simulink model "twoarealfc"  (R2025a)
settings: Solver=VariableStepAuto  StartTime=0.0  StopTime=10  RelTol=1e-3
settings Model: Creator=Lijoofficial  LastModifiedBy=Lijoofficial

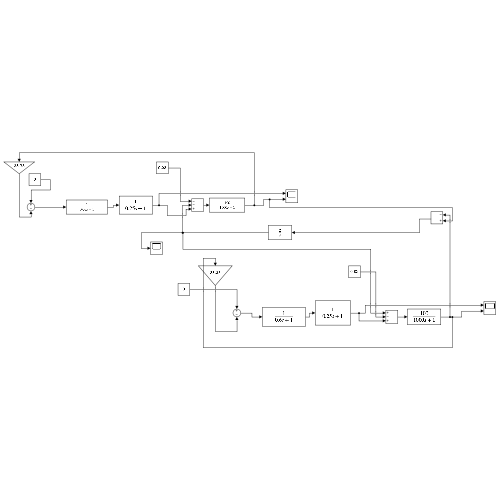
[thumbnail: Simulink's stored preview of the top-level diagram]
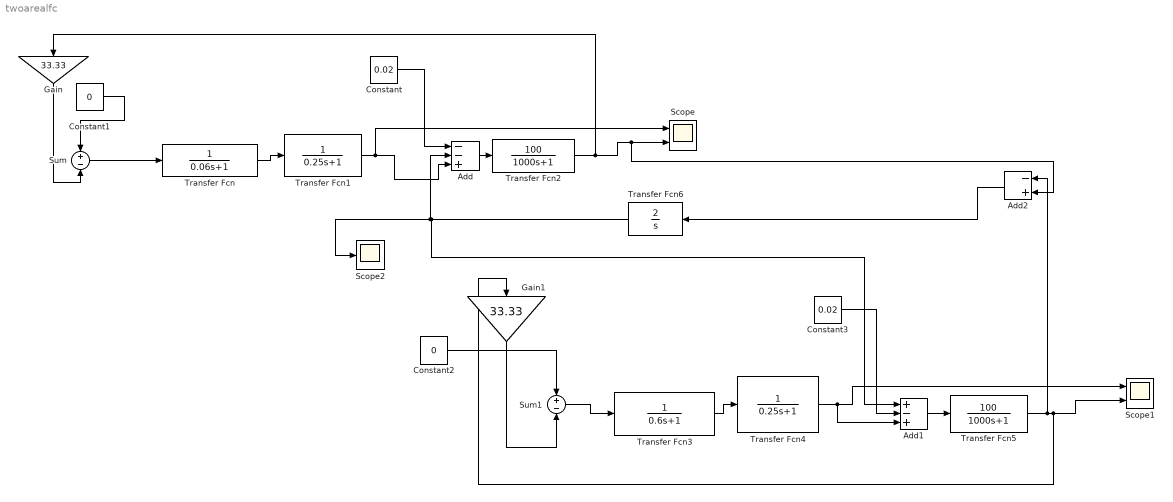
== system twoarealfc ==
  Add : Sum  Inputs=--+
  Add1 : Sum  Inputs=+-+
  Add2 : Sum  Inputs=-+
  Constant : Constant  Value=0.02
  Constant1 : Constant  Value=0
  Constant2 : Constant  Value=0
  Constant3 : Constant  Value=0.02
  Gain : Gain  Gain=33.33
  Gain1 : Gain  Gain=33.33
  Scope : Scope  NumInputPorts=2
      settings: ActiveDisplayYMinimum=-0.0030308251312968744  ActiveDisplayYMaximum=0.027277426181671879
  Scope1 : Scope  NumInputPorts=2
      settings: ActiveDisplayYMinimum=-0.0040459045659060281  ActiveDisplayYMaximum=0.036413141093154258
  Scope2 : Scope
      settings: ActiveDisplayYMinimum=-0.0001454427191426443  ActiveDisplayYMaximum=0.0012648016775742409  DataLoggingVariableName=ScopeData2
  Sum : Sum  Inputs=+-
  Sum1 : Sum  Inputs=+-
  Transfer Fcn : TransferFcn  Denominator=[0.06 1]
  Transfer Fcn1 : TransferFcn  Denominator=[0.25 1]
  Transfer Fcn2 : TransferFcn  Numerator=100  Denominator=[1000 1]
  Transfer Fcn3 : TransferFcn  Denominator=[0.6 1]
  Transfer Fcn4 : TransferFcn  Denominator=[0.25 1]
  Transfer Fcn5 : TransferFcn  Numerator=100  Denominator=[1000 1]
  Transfer Fcn6 : TransferFcn  Numerator=2  Denominator=[1 0]
  wires:
  Transfer Fcn/1 -> Transfer Fcn1/1
  Transfer Fcn1/1 -> Scope/1, Add/3
  Add/1 -> Transfer Fcn2/1
  Constant/1 -> Add/1
  Transfer Fcn2/1 -> Gain/1, Add2/2, Scope/2
  Transfer Fcn5/1 -> Add2/1, Gain1/1, Scope1/2
  Transfer Fcn4/1 -> Add1/3, Scope1/1
  Add1/1 -> Transfer Fcn5/1
  Transfer Fcn3/1 -> Transfer Fcn4/1
  Add2/1 -> Transfer Fcn6/1
  Transfer Fcn6/1 -> Add1/1, Add/2, Scope2/1
  Gain/1 -> Sum/2
  Sum/1 -> Transfer Fcn/1
  Constant1/1 -> Sum/1
  Constant2/1 -> Sum1/1
  Gain1/1 -> Sum1/2
  Sum1/1 -> Transfer Fcn3/1
  Constant3/1 -> Add1/2
